simulink model "Mech_sys_nl_obs"  (R2025b)
settings: Solver=ode15s  StartTime=0.0  StopTime=28  RelTol=1e-3
values from neighbouring files (symbols this model uses):
  p_0 = 0    [Init_Simulink_param.m]
  phat_0 = 1e-3    (= 0.001)    [Init_Simulink_param.m]
  q_0 = 0    [Init_Simulink_param.m]
  qhat_0 = 2e-4    (= 0.0002)    [Init_Simulink_param.m]
undefined symbols (not defined in the file or in its folder): params
libraries: simulink x1
settings Model: Creator=filippougolini  LastModifiedBy=filippougolini

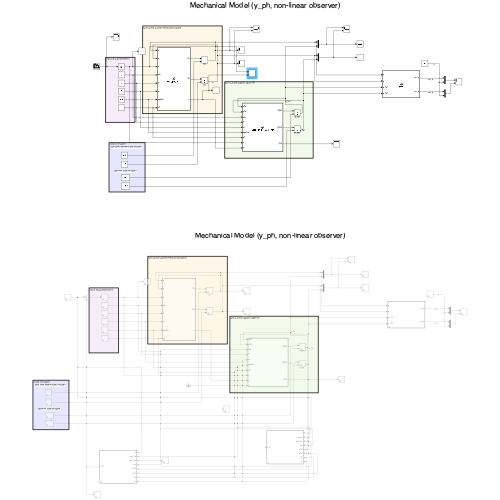
[thumbnail: Simulink's stored preview of the top-level diagram]
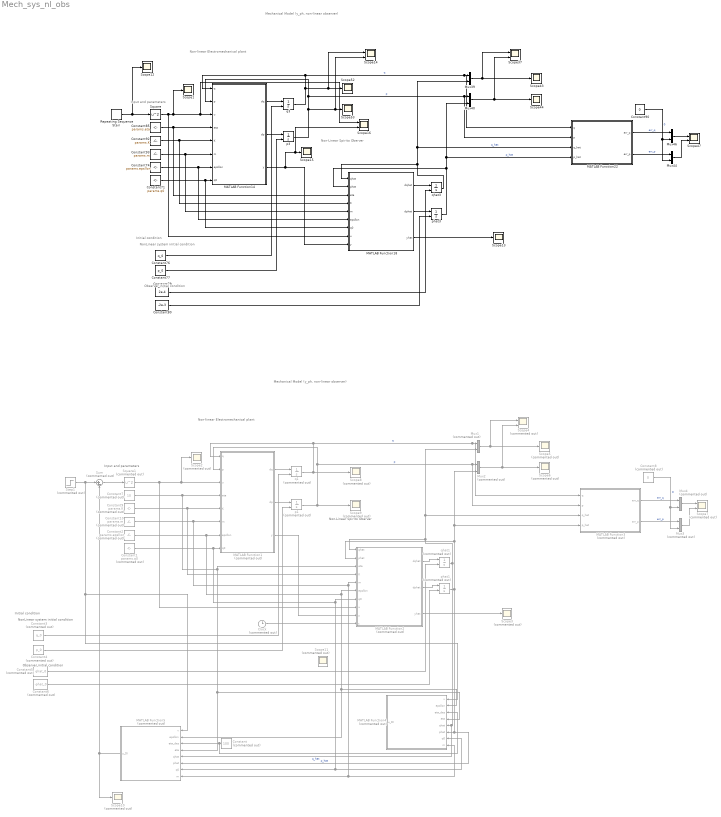
== system Mech_sys_nl_obs ==
  note: Mechanical Model (y_ph, non-linear observer)
  note: Initial condition
  note: Input and parameters
  note: Non-linear Electromechanical plant
  note: Observer initial condition
  note: NonLinear system initial condition
  note: Non-Linear Spirito Oberver
  note: Non-Linear Spirito Oberver
  note: NonLinear system initial condition
  note: Input and parameters
  note: Mechanical Model (y_ph, non-linear observer)
  note: Initial condition
  note: Non-linear Electromechanical plant
  note: Observer initial condition
  Clock : Clock  Commented=on
  Constant : Constant  Commented=on  Value=100
  Constant1 : Constant  Commented=on  Value=params.q0
  Constant10 : Constant  Commented=on  Value=params.m
  Constant2 : Constant  Commented=on  Value=params.epsllon
  Constant3 : Constant  Commented=on  Value=q_0
  Constant4 : Constant  Commented=on  Value=p_0
  Constant5 : Constant  Commented=on  Value=qhat_0
  Constant6 : Constant  Commented=on  Value=-phat_0
  Constant7 : Constant  Commented=on  Value=10
  Constant71 : Constant  Value=params.q0
  Constant74 : Constant  Value=params.epsllon
  Constant76 : Constant  Value=q_0
  Constant77 : Constant  Value=p_0
  Constant79 : Constant  Value=2e-4
  Constant8 : Constant  Commented=on  Value=0
  Constant80 : Constant  Value=-2e-3
  Constant85 : Constant  Value=params.eta
  Constant9 : Constant  Commented=on  Value=params.K
  Constant90 : Constant  Value=0
  Constant92 : Constant  Value=params.K
  Constant93 : Constant  Value=params.m
  MATLAB Function1 : MATLAB Function  Commented=on  TreatAsAtomicUnit=on
  MATLAB Function14 : MATLAB Function  TreatAsAtomicUnit=on
  MATLAB Function18 : MATLAB Function  TreatAsAtomicUnit=on
  MATLAB Function2 : MATLAB Function  Commented=on  TreatAsAtomicUnit=on
  MATLAB Function22 : MATLAB Function  TreatAsAtomicUnit=on
  MATLAB Function3 : MATLAB Function  Commented=on  TreatAsAtomicUnit=on
  MATLAB Function4 : MATLAB Function  Commented=on  TreatAsAtomicUnit=on
  MATLAB Function5 : MATLAB Function  Commented=on  TreatAsAtomicUnit=on
  Mux{1..4} (4 alike) : Mux  Commented=on  Inputs=2
  Mux{39..40,44,46} (4 alike) : Mux  Inputs=2
  Repeating Sequence Stair : simulink/Sources/Repeating Sequence Stair  OutValues=[0 5000 4000 2000 4000 3000 0].'  tsamp=4  OutMin=[]  OutMax=[]  OutDataTypeStr=double  OutputDataTypeScalingMode=double  OutDataType=fixdt(0,8)  ConRadixGroup=Best Precision: Vector-wise  OutScaling=2^-12
  Scope{1,12..13,15,43..44,52..53} (8 alike) : Scope
      Scope1 settings: ActiveDisplayYMinimum=-1  ActiveDisplayYMaximum=1
      Scope12 settings: ActiveDisplayYMinimum=-1  ActiveDisplayYMaximum=1  DataLoggingVariableName=ScopeData11
      Scope13 settings: ActiveDisplayYMinimum=999.83794210721385  ActiveDisplayYMaximum=1000.4797286758781  DataLoggingVariableName=ScopeData12
      Scope15 settings: ActiveDisplayYMinimum=-2.5338402834634636E-11  ActiveDisplayYMaximum=1.9121817917651133E-11  DataLoggingVariableName=ScopeData14
      Scope43 settings: ActiveDisplayYMinimum=-4.4929456410290065E-5  ActiveDisplayYMaximum=0.00036894675529116814  DataLoggingVariableName=ScopeData43
      Scope44 settings: ActiveDisplayYMinimum=-1  ActiveDisplayYMaximum=1  DataLoggingVariableName=ScopeData44
      Scope52 settings: ActiveDisplayYMinimum=-4.0944874698701246E-5  ActiveDisplayYMaximum=0.0003685038722883113  DataLoggingVariableName=ScopeData52
      Scope53 settings: ActiveDisplayYMinimum=-1  ActiveDisplayYMaximum=1  DataLoggingVariableName=ScopeData53
  Scope{2..3,5..6,8..11} (8 alike) : Scope  Commented=on
      Scope10 settings: ActiveDisplayYMinimum=-1  ActiveDisplayYMaximum=1  DataLoggingVariableName=ScopeData9
      Scope11 settings: ActiveDisplayYMinimum=-279.84500015647927  ActiveDisplayYMaximum=2334.0816420191145  DataLoggingVariableName=ScopeData10
      Scope2 settings: ActiveDisplayYMinimum=-1  ActiveDisplayYMaximum=1
      Scope3 settings: ActiveDisplayYMinimum=999.83794210721385  ActiveDisplayYMaximum=1000.4797286758781  DataLoggingVariableName=ScopeData2
      Scope5 settings: ActiveDisplayYMinimum=-4.4929456410290065E-5  ActiveDisplayYMaximum=0.00036894675529116814  DataLoggingVariableName=ScopeData4
      Scope6 settings: ActiveDisplayYMinimum=-1  ActiveDisplayYMaximum=1  DataLoggingVariableName=ScopeData5
      Scope8 settings: ActiveDisplayYMinimum=-4.0944874698701246E-5  ActiveDisplayYMaximum=0.0003685038722883113  DataLoggingVariableName=ScopeData7
      Scope9 settings: ActiveDisplayYMinimum=-1  ActiveDisplayYMaximum=1  DataLoggingVariableName=ScopeData8
  Scope{14,16,37,47} (4 alike) : Scope  NumInputPorts=2
      Scope14 settings: ActiveDisplayYMinimum=-0.0073723529835781629  ActiveDisplayYMaximum=0.0032936654175013554  DataLoggingVariableName=ScopeData13
      Scope16 settings: ActiveDisplayYMinimum=-2.5338402834634636E-11  ActiveDisplayYMaximum=1.9121817917651133E-11  DataLoggingVariableName=ScopeData15
      Scope37 settings: ActiveDisplayYMinimum=-0.0073528020829721329  ActiveDisplayYMaximum=0.0032925360279497883  DataLoggingVariableName=ScopeData37
      Scope47 settings: ActiveDisplayYMinimum=-9.9731359660129417E-14  ActiveDisplayYMaximum=8.2901053967544525E-14  DataLoggingVariableName=ScopeData47
  Scope4 : Scope  Commented=on  NumInputPorts=2
      settings: ActiveDisplayYMinimum=-0.0044230014521020418  ActiveDisplayYMaximum=0.0021122811902405379  DataLoggingVariableName=ScopeData3
  Scope7 : Scope  Commented=on  NumInputPorts=2
      settings: ActiveDisplayYMinimum=-0.0018731640888278536  ActiveDisplayYMaximum=0.00439643288527841  DataLoggingVariableName=ScopeData6
  Square : Math  Operator=square
  Square1 : Math  Commented=on  Operator=square
  Step1 : Step  Commented=on  After=5e3  SampleTime=0
  Sum : Sum  Commented=on  Inputs=|+-
  p1 : Integrator  Commented=on  InitialConditionSource=external
  p3 : Integrator  InitialConditionSource=external
  phat1 : Integrator  Commented=on  InitialConditionSource=external  InitialCondition=5e-4
  phat3 : Integrator  InitialConditionSource=external  InitialCondition=5e-4
  q1 : Integrator  Commented=on  InitialConditionSource=external
  q3 : Integrator  InitialConditionSource=external
  qhat1 : Integrator  Commented=on  InitialConditionSource=external  InitialCondition=20e-5
  qhat3 : Integrator  InitialConditionSource=external  InitialCondition=20e-5
  wires:
  MATLAB Function18/1(dqhat) -> qhat3/1
  Mux39/1 -> Scope37/1, Scope43/1
  Mux44/1 -> Scope47/2
  Constant77/1 -> p3/2
  Constant76/1 -> q3/2
  q3/1 -> Scope14/1, Scope52/1, Mux39/1, MATLAB Function22/1(q), MATLAB Function14/1(q)  "q"
  Constant92/1 -> MATLAB Function18/4(K), MATLAB Function14/5(K)
  Constant85/1 -> MATLAB Function18/3(eta), MATLAB Function14/4(eta)
  Constant79/1 -> qhat3/2
  p3/1 -> Scope14/2, Scope53/1, Mux40/1, MATLAB Function22/2(p), MATLAB Function14/2(p)  "p"
  MATLAB Function22/1(err_q) -> Mux46/1  "err_q"
  Constant90/1 -> Mux44/2, Mux46/2  "0"
  Constant80/1 -> phat3/2
  MATLAB Function18/2(dphat) -> phat3/1
  MATLAB Function22/2(err_p) -> Mux44/1  "err_p"
  MATLAB Function14/1(dq) -> q3/1
  Constant74/1 -> MATLAB Function18/6(epsllon), MATLAB Function14/7(epsllon)
  MATLAB Function18/3(yhat) -> Scope13/1
  qhat3/1 -> Mux39/2, MATLAB Function22/3(q_hat), MATLAB Function18/1(qhat)  "q_hat"
  Mux40/1 -> Scope37/2, Scope44/1
  Constant71/1 -> MATLAB Function18/7(q0), MATLAB Function14/8(q0)
  Constant93/1 -> MATLAB Function18/5(m), MATLAB Function14/6(m)
  Mux46/1 -> Scope47/1
  phat3/1 -> Mux40/2, MATLAB Function22/4(p_hat), MATLAB Function18/2(phat)  "p_hat"
  MATLAB Function14/2(dp) -> p3/1
  Repeating Sequence Stair/1 -> Scope12/1, Square/1
  Square/1 -> Scope16/1, MATLAB Function14/3(u), Scope1/1, MATLAB Function18/8(u)
  Mux3/1 -> Scope7/2
  Constant3/1 -> q1/2
  Constant1/1 -> MATLAB Function4/7(q0), MATLAB Function5/7(q0), MATLAB Function2/7(q0), MATLAB Function1/8(q0)
  Constant9/1 -> MATLAB Function2/4(K), MATLAB Function1/5(K)
  Constant10/1 -> MATLAB Function4/8(m), MATLAB Function5/8(m), MATLAB Function2/5(m), MATLAB Function1/6(m)
  MATLAB Function1/1(dq) -> q1/1
  Constant2/1 -> MATLAB Function5/2(epsllon), MATLAB Function4/2(epsllon), MATLAB Function2/6(epsllon), MATLAB Function1/7(epsllon)
  Mux2/1 -> Scope4/2, Scope6/1
  MATLAB Function2/2(dphat) -> phat1/1
  phat1/1 -> MATLAB Function4/6(phat), MATLAB Function5/6(phat), Mux2/2, MATLAB Function3/4(p_hat), MATLAB Function2/2(phat)  "p_hat"
  Constant6/1 -> phat1/2
  MATLAB Function3/1(err_q) -> Mux4/1  "err_q"
  MATLAB Function2/1(dqhat) -> qhat1/1
  Constant5/1 -> qhat1/2
  Constant8/1 -> Mux3/2, Mux4/2  "0"
  Constant7/1 -> MATLAB Function2/3(eta), MATLAB Function5/4(eta), MATLAB Function4/4(eta), MATLAB Function1/4(eta)
  q1/1 -> Mux1/1, MATLAB Function3/1(q), MATLAB Function1/1(q), Scope8/1  "q"
  MATLAB Function1/3(y) -> MATLAB Function2/9(y)
  MATLAB Function1/2(dp) -> p1/1
  Constant4/1 -> p1/2
  p1/1 -> Mux2/1, MATLAB Function3/2(p), MATLAB Function1/2(p), Scope9/1  "p"
  Mux4/1 -> Scope7/1
  Mux1/1 -> Scope4/1, Scope5/1
  MATLAB Function2/3(yhat) -> Scope3/1
  MATLAB Function3/2(err_p) -> Mux3/1  "err_p"
  qhat1/1 -> Mux1/2, MATLAB Function3/3(q_hat), MATLAB Function2/1(qhat), MATLAB Function5/5(qhat), MATLAB Function4/5(qhat)  "q_hat"
  Sum/1 -> Square1/1
  MATLAB Function5/1(u_DI) -> Sum/2, Scope10/1
  Constant/1 -> MATLAB Function4/3(eta_des), MATLAB Function5/3(eta_des)
  Step1/1 -> MATLAB Function4/1(v), MATLAB Function5/1(v), Sum/1
  Square1/1 -> MATLAB Function2/8(u), MATLAB Function1/3(u), Scope2/1
  Clock/1 -> MATLAB Function2/10(t)
  MATLAB Function14/3(y) -> MATLAB Function18/9(y), Scope16/2, Scope15/1

== matlab function Mech_sys_nl_obs/MATLAB Function18 ==
  data: qhat input; phat input; eta input; K input; m input; epsllon input; q0 input; u input; dqhat output; y input; dphat output; yhat output
function [dqhat, dphat, yhat] = observer_pH_mech_yph(qhat, phat, ...
    eta, K, m, epsllon, q0, u, y)

    % Port-Hamiltonian structure matrices
    J = [  0  1;
          -1  0 ];

    R = diag([0, eta]);
    g = [0; 2*epsllon*(qhat + q0)^3];

    % dH/dqhat
    dHhdqh = K*qhat;
    % dH/dphat
    dHhdph = phat / m;
    % dH/dQhat

    gradHh = [dHhdqh; dHhdph];
    L = [0, 20*2*epsllon*(qhat + q0)^3];

    % L = 1.0e+06 * [-0.0657, 3.1779];

    % --------Observer gain L --------
    Lcol = L.';       % ensure it's 3x1

    yhat = 2*(phat / m)*epsllon*(qhat + q0)^3;

    % -------- Observer dynamics --------
    % Note: J and R are constant
    xhatdot = (J - R) * gradHh + g*u + Lcol * (y - yhat);

    dqhat = xhatdot(1);
    dphat = xhatdot(2);
end

== matlab function Mech_sys_nl_obs/MATLAB Function22 ==
  data: q input; err_q output; p input; q_hat input; p_hat input; err_p output
function [err_q, err_p] = error(q, p, q_hat, p_hat)

    err_q = q - q_hat;
    err_p = p - p_hat;
end

== matlab function Mech_sys_nl_obs/MATLAB Function1 ==
  data: q input; p input; u input; dq output; eta input; K input; m input; epsllon input; q0 input; dp output; y output
function [dq, dp, y] = plant_pH_mech(q, p, u, eta, K, m, epsllon, q0)
% Electro-mechanical pH plant

    % Parameters: m, K, eta, eps, re, q0 in workspace

    J = [  0  1 ;
          -1  0 ];

    R = diag([0, eta]);
    g = [0; 2*epsllon*(q + q0)^3];

    dHdq = K * q;
    dHdp = p / m;

    gradH = [dHdq; dHdp];

    xdot = (J - R) * gradH + g*u;

    y = 2*(p / m)*epsllon*(q + q0)^3;

    
    dq = xdot(1);
    dp = xdot(2);
end

== matlab function Mech_sys_nl_obs/MATLAB Function2 ==
  data: qhat input; phat input; eta input; K input; m input; epsllon input; q0 input; u input; dqhat output; y input; dphat output; yhat output; t input
function [dqhat, dphat, yhat] = observer_pH_mech_yph(qhat, phat, ...
    eta, K, m, epsllon, q0, u, y, t)

    % Port-Hamiltonian structure matrices
    J = [  0  1;
          -1  0 ];

    R = diag([0, eta]);
    g = [0; 2*epsllon*(qhat + q0)^3];

    % dH/dqhat
    dHhdqh = K*qhat;
    % dH/dphat
    dHhdph = phat / m;
    % dH/dQhat

    gradHh = [dHhdqh; dHhdph];

    yhat = 2*(phat / m)*epsllon*(qhat + q0)^3;
    % L = [0, 20*2*epsllon*(qhat + q0)^3];
    % after computing yhat
    ey = y - yhat;
    
    % --- gain scheduling parameters ---
    if t <=1
        l2 = 2000000000;
    else
        l2 = 20;
    end
    L = [0 l2];

    % -------- Observer gain L --------
    Lcol = L.';       % ensure it's 3x1


    % -------- Observer dynamics --------
    % Note: J and R are constant
    xhatdot = (J - R) * gradHh + g*u + Lcol * (y - yhat);

    dqhat = xhatdot(1);
    dphat = xhatdot(2);
end

== matlab function Mech_sys_nl_obs/MATLAB Function3 ==
  data: q input; err_q output; p input; q_hat input; p_hat input; err_p output
function [err_q, err_p] = error(q, p, q_hat, p_hat)

    err_q = q - q_hat;
    err_p = p - p_hat;
end

== matlab function Mech_sys_nl_obs/MATLAB Function4 ==
  data: v input; u_DI output; epsllon input; eta_des input; eta input; qhat input; phat input; q0 input; m input
function u_DI = fcn(v, epsllon, eta_des, eta, qhat, phat, q0, m)
%#codegen

v_min  = 0.05;
p_min  = 1e-6;

% measurement-like signal
y = 2*(phat/m)*epsllon*(qhat + q0)^3;

% ---- Always initialize for codegen ----
Kd_0 = 0;

% Compute Kd_0 for the v≈0 branch (your idea)
alpha9 = (qhat + q0)^9;

num = (-eta_des + eta + 2*20*epsllon*(qhat + q0)^3);
den = (4*epsllon^2*alpha9);

% Avoid division by zero
if abs(den) < 1e-12
    den = 1e-12;
end

% Use abs(phat) (you had a sign split; abs is simpler and coder-friendly)
p_use = abs(phat);
if p_use < p_min
    p_use = p_min;
end

rad = (num/den) * (p_use/m);

% Prevent complex sqrt
if rad < 0
    rad = 0;
end

Kd_0 = sqrt(rad);

% ---- If v is too small: use Kd_0 and sign like you wanted ----
if abs(v) < v_min
    if phat >= 0
        u_DI =  Kd_0 * y;
    else
        u_DI = -Kd_0 * y;
    end
    return;
end

% ---- Otherwise: your quadratic/linear logic ----
alpha6 = (qhat + q0)^6;

a = 8*(epsllon^3)*alpha9*(phat/m);
b = -8*(epsllon^2)*alpha6*v;
c = (eta_des - eta);

% Default Kd
Kd = 0;

% If a ~ 0 -> linear fallback
if abs(phat) < p_min || abs(a) < 1e-12
    Kd = (eta_des - eta) / (8*epsllon^2*alpha6*v);
else
    disc = b*b - 4*a*c;

    if disc < 0
        % fallback
        Kd = (eta_des - eta) / (8*epsllon^2*alpha6*v);
    else
        sqrt_disc = sqrt(disc);

        Kd1 = (-b + sqrt_disc) / (2*a);
        Kd2 = (-b - sqrt_disc) / (2*a);

        ok1 = isfinite(Kd1) && (Kd1 >= 0);
        ok2 = isfinite(Kd2) && (Kd2 >= 0);

        if ok1 && ok2
            Kd = min(Kd1, Kd2);
        elseif ok1
            Kd = Kd1;
        elseif ok2
            Kd = Kd2;
        else
            Kd = (eta_des - eta) / (8*epsllon^2*alpha6*v);
        end
    end
end

% Enforce finite / real (and nonnegative if you want)
if ~isfinite(Kd) || ~isreal(Kd)
    Kd = 0;
end
% If you want to allow negative Kd, comment this out
if Kd < 0
    Kd = 0;
end

u_DI = Kd * y;

end

== matlab function Mech_sys_nl_obs/MATLAB Function5 ==
  data: v input; u_DI output; epsllon input; eta_des input; eta input; qhat input; phat input; q0 input; m input
function u_DI = fcn(v, epsllon, eta_des, eta, qhat, phat, q0, m)
    y_hat = 2*epsllon*(phat/m)*(qhat + q0)^3;
    v_min = 0.05;
    if v < v_min
        Kd = 0;
    else
        Kd = (eta_des - eta)/(8*epsllon^2*(qhat + q0)^6*v);
    end
    u_DI = Kd * y_hat;
end

== matlab function Mech_sys_nl_obs/MATLAB Function14 ==
  data: q input; p input; u input; dq output; eta input; K input; m input; epsllon input; q0 input; dp output; y output
function [dq, dp, y] = plant_pH_mech(q, p, u, eta, K, m, epsllon, q0)
% Electro-mechanical pH plant

    % Parameters: m, K, eta, eps, re, q0 in workspace

    J = [  0  1 ;
          -1  0 ];

    R = diag([0, eta]);
    g = [0; 2*epsllon*(q + q0)^3];

    dHdq = K * q;
    dHdp = p / m;

    gradH = [dHdq; dHdp];

    xdot = (J - R) * gradH + g*u;

    y = 2*(p / m)*epsllon*(q + q0)^3;

    
    dq = xdot(1);
    dp = xdot(2);
end
